simulink model "intgratedMCUSlugs"  (Simulink 7.8)
settings: Solver=FixedStepDiscrete  SolverMode=SingleTasking  StartTime=0.0  StopTime=10.0  FixedStep=0.001  RelTol=1e-3
InitFcn:
  | mcuInit
undefined symbols (not defined in the file): accBiasRateLimit, apSampleTime, barAdjust, baroCutoff, baroCutTemp, baroOffset, baroScale, barTGain1, barTGain2, barTMean1, barTMean2, baseHeight, baseTemp, bda, bde, bdr, bdt, bICda, bICde, bICdr, bICdt, bpan, bPWMpan, bPWMtilt, broll, btilt, changeZoom, controlMCUInit, cubeAccelGain16405, cubeGyroGain16405, cubeMagGain16405, daTrimMax, daTrimMin, deTrimMax, deTrimMin, DiscIntNeverNeededParam, drTrimMax, drTrimMin, dtTrimMax, dtTrimMin, Function_Update, gaind, getCubeData, getGpsMainData, getGPSRawData, getGpsUbloxMainData, getGSLocation, getISRLocation, getMidLevelCommands, getMobileLocation, getPassValues, getRangeOfParams, getRTB, gpsParse, gsRead, gyroBiasRateLimit, hil_getEuler, hil_getRates, hil_getRawRead, hil_getVned ... (+89)
libraries: dsPICdrivers x105, simulink x14, SLUGS_Library x12, aerolibconvert2 x5, aerolibutil x4, aerolibtransform2 x3, dspmtrx3 x3, aerolibobsolete x3
(part 4 of 6)

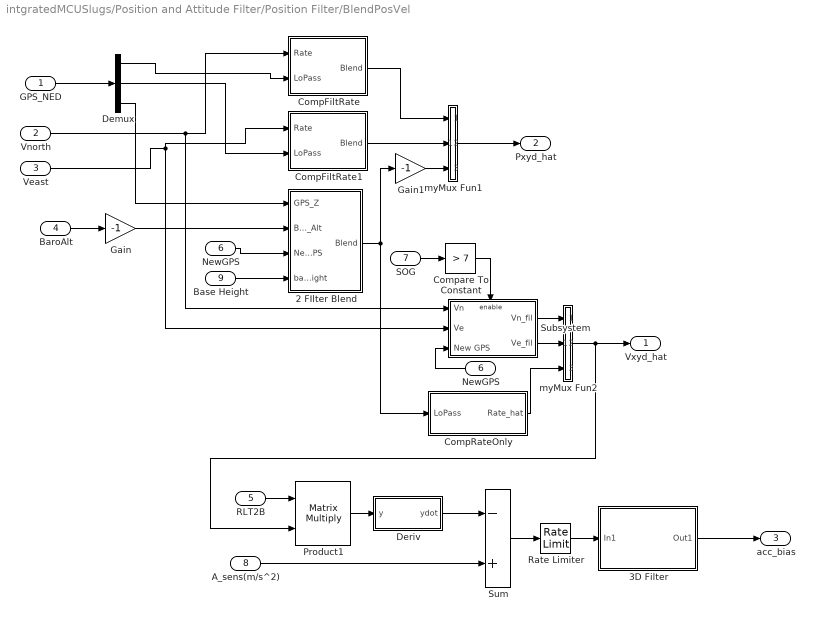
== system intgratedMCUSlugs/Position and Attitude Filter/Position Filter/BlendPosVel ==
  GPS_NED : Inport
  Vnorth : Inport  Port=2
  Veast : Inport  Port=3
  BaroAlt : Inport  Port=4
  RLT2B : Inport  Port=5
  NewGPS : Inport  Port=6
  SOG : Inport  Port=7
  A_sens(m/s^2) : Inport  Port=8
  Base Height : Inport  Port=9
  2 FIlter Blend : Subsystem
  3D Filter : Subsystem  AncestorBlock=SLUGS_Library/Singnal Routing & Conditioning/3D Filter  RTWFcnName=TustinFilter3D  mask{zval=[], pval=-1/accBiasRateLimit, kval=1, TSample=0.01}
      mask prompts: zval "Zeros"; pval "Poles"; kval "Gains"; TSample "Sample Time"
      settings: RTWFcnNameOpts=User specified  RTWFileNameOpts=Use function name
      mask Display:
      | droots(zval,pval,kval)
      | port_label('input',1,'3D')
  CompFiltRate : Subsystem  mask{omega=xCutoff, T=apSampleTime}
      mask prompts: omega "Cutoff Freq (rad/sec)"; T "Sample Time"
  CompFiltRate1 : Subsystem  mask{omega=yCutoff, T=apSampleTime}
      mask prompts: omega "Cutoff Freq (rad/sec)"; T "Sample Time"
  CompRateOnly : Subsystem  mask{omega=vzCutoff, T=apSampleTime}
      mask prompts: omega "Cutoff Freq (rad/sec)"; T "Sample Time"
  Compare To Constant : simulink/Logic and Bit Operations/Compare To Constant  relop=>  const=7  OutDataTypeStr=uint8  ZeroCross=off
  Demux : Demux  Outputs=3
  "Deriv " : Subsystem
  Gain : Gain  Gain=-1
  Gain1 : Gain  Gain=-1  OutDataTypeStr=Inherit: Same as input
  "NewGPS " : InportShadow  Port=6
  Product1 : Product  Multiplication=Matrix(*)  RndMeth=Zero
  Rate Limiter : RateLimiter  RisingSlewLimit=accBiasRateLimit  FallingSlewLimit=-accBiasRateLimit  SampleTimeMode=inherited
  Subsystem : Subsystem
  Sum : Sum  Inputs=-+  OutDataTypeStr=single
  myMux Fun1 : MATLAB Function  TreatAsAtomicUnit=on
  myMux Fun2 : MATLAB Function  TreatAsAtomicUnit=on
  Vxyd_hat : Outport
  Pxyd_hat : Outport  Port=2
  acc_bias : Outport  Port=3
  wires:
  CompRateOnly/1(Rate_hat) -> myMux Fun2/3(u3)
  Subsystem/2(Ve_fil) -> myMux Fun2/2(u2)
  Subsystem/1(Vn_fil) -> myMux Fun2/1(u1)
  myMux Fun1/1(y) -> Pxyd_hat/1
  2 FIlter Blend/1(Blend) -> Gain1/1, CompRateOnly/1(LoPass)
  CompFiltRate/1(Blend) -> myMux Fun1/1(u1)
  CompFiltRate1/1(Blend) -> myMux Fun1/2(u2)
  Demux/3 -> 2 FIlter Blend/1(GPS_Z)
  BaroAlt/1 -> Gain/1
  Demux/2 -> CompFiltRate1/2(LoPass)
  Demux/1 -> CompFiltRate/2(LoPass)
  Veast/1 -> CompFiltRate1/1(Rate), Subsystem/2(Ve)
  Vnorth/1 -> Subsystem/1(Vn), CompFiltRate/1(Rate)
  GPS_NED/1 -> Demux/1
  Gain1/1 -> myMux Fun1/3(u3)
  myMux Fun2/1(y) -> Vxyd_hat/1, Product1/2
  NewGPS/1 -> Subsystem/3(New GPS)
  Compare To Constant/1 -> Subsystem/Enable
  SOG/1 -> Compare To Constant/1
  Rate Limiter/1 -> 3D Filter/1(In1)
  3D Filter/1(Out1) -> acc_bias/1
  Sum/1 -> Rate Limiter/1
  Product1/1 -> "Deriv "/1(y)
  "Deriv "/1(ydot) -> Sum/1
  A_sens(m/s^2)/1 -> Sum/2
  RLT2B/1 -> Product1/1
  Gain/1 -> 2 FIlter Blend/2(Baro_Alt)
  "NewGPS "/1 -> 2 FIlter Blend/3(New GPS)
  Base Height/1 -> 2 FIlter Blend/4(baseHeight)

== system intgratedMCUSlugs/Sensor Data/Sensor Suite/ADIS16405 Signal Cond  ==
  Gyro Raw : Inport
  Accel Raw : Inport  Port=2
  Mag Raw : Inport  Port=3
  "3D Tustin Lowpass, Auto Initial Condition" : Subsystem  mask(Tustin1stOrderLowpassAutoInitialCondition){f=mainSensorCutoff, T=T}
      mask prompts: f "Lowpass Frequency"; T "Sample Time"
      mask help: Takes a 3db rolloff frequency (in Hz, NOT radians/s) and a sample time. Performs a symbolic Tustin conversion and implements in a discrete filter. The initial output of the filter is set by the first sample.
      mask Help: Enter the desired 3db rolloff frequency in Hz and the sample time. Initial conditions are sampled automatically.
      mask Display: fprintf('%.2f Hz lowpass (3D)',f)
  "3D Tustin Lowpass, Auto Initial Condition1" : Subsystem  mask(Tustin1stOrderLowpassAutoInitialCondition){f=mainSensorCutoff, T=T}
      mask prompts: f "Lowpass Frequency"; T "Sample Time"
      mask help: Takes a 3db rolloff frequency (in Hz, NOT radians/s) and a sample time. Performs a symbolic Tustin conversion and implements in a discrete filter. The initial output of the filter is set by the first sample.
      mask Help: Enter the desired 3db rolloff frequency in Hz and the sample time. Initial conditions are sampled automatically.
      mask Display: fprintf('%.2f Hz lowpass (3D)',f)
  "3D Tustin Lowpass, Auto Initial Condition2" : Subsystem  mask(Tustin1stOrderLowpassAutoInitialCondition){f=mainSensorCutoff, T=T}
      mask prompts: f "Lowpass Frequency"; T "Sample Time"
      mask help: Takes a 3db rolloff frequency (in Hz, NOT radians/s) and a sample time. Performs a symbolic Tustin conversion and implements in a discrete filter. The initial output of the filter is set by the first sample.
      mask Help: Enter the desired 3db rolloff frequency in Hz and the sample time. Initial conditions are sampled automatically.
      mask Display: fprintf('%.2f Hz lowpass (3D)',f)
  Data Type Conversion1 : DataTypeConversion  OutDataTypeStr=double
  Data Type Conversion2 : DataTypeConversion  OutDataTypeStr=double
  Data Type Conversion3 : DataTypeConversion  OutDataTypeStr=single
  Data Type Conversion5 : DataTypeConversion  OutDataTypeStr=double
  Data Type Conversion6 : DataTypeConversion  OutDataTypeStr=single
  Data Type Conversion7 : DataTypeConversion  OutDataTypeStr=single
  Divide : Product  OutDataTypeStr=single
  Divide1 : Product  OutDataTypeStr=single
  Divide2 : Product  OutDataTypeStr=single
  Gyro Gains : Constant  Value=cubeGyroGain16405  OutDataTypeStr=single
  Gyro Gains1 : Constant  Value=cubeAccelGain16405  OutDataTypeStr=single
  Gyro Gains2 : Constant  Value=cubeMagGain16405  OutDataTypeStr=single
  Rotate Cube Axis : Subsystem
  "Rotate Cube Axis " : Subsystem
  "Rotate Cube Axis  " : Subsystem
  Omega (rad/s) : Outport
  Accel (m/s^2) : Outport  Port=2
  Mags (mG) : Outport  Port=3
  wires:
  Gyro Gains/1 -> Divide/2
  Divide/1 -> Rotate Cube Axis/1(Raw)
  Divide1/1 -> "Rotate Cube Axis "/1(Raw)
  "Rotate Cube Axis "/1(Rotated) -> Data Type Conversion1/1
  Gyro Gains1/1 -> Divide1/2
  Gyro Raw/1 -> Divide/1
  Data Type Conversion2/1 -> "3D Tustin Lowpass, Auto Initial Condition"/1(In1)
  "3D Tustin Lowpass, Auto Initial Condition"/1(Out1) -> Data Type Conversion7/1
  Data Type Conversion7/1 -> Omega (rad/s)/1
  Rotate Cube Axis/1(Rotated) -> Data Type Conversion2/1
  Data Type Conversion1/1 -> "3D Tustin Lowpass, Auto Initial Condition1"/1(In1)
  "3D Tustin Lowpass, Auto Initial Condition1"/1(Out1) -> Data Type Conversion3/1
  Data Type Conversion3/1 -> Accel (m/s^2)/1
  Accel Raw/1 -> Divide1/1
  Divide2/1 -> "Rotate Cube Axis  "/1(Raw)
  Data Type Conversion5/1 -> "3D Tustin Lowpass, Auto Initial Condition2"/1(In1)
  "3D Tustin Lowpass, Auto Initial Condition2"/1(Out1) -> Data Type Conversion6/1
  Data Type Conversion6/1 -> Mags (mG)/1
  "Rotate Cube Axis  "/1(Rotated) -> Data Type Conversion5/1
  Mag Raw/1 -> Divide2/1
  Gyro Gains2/1 -> Divide2/2

== system intgratedMCUSlugs/Sensor Data/Sensor Suite/Compute CPU Load ==
  Calculus Time Step : dsPICdrivers/OTHERS/Calculus Time Step  Tag=dsPIC_CalculusTimeStep  SampleTime=0.01  PR1chk=on
  Constant : Constant
  Data Type Conversion1 : DataTypeConversion  OutDataTypeStr=single
  Data Type Conversion12 : DataTypeConversion  OutDataTypeStr=uint8
  Data Type Conversion2 : DataTypeConversion  OutDataTypeStr=single
  Divide : Product  Inputs=*/  OutDataTypeStr=double
  Gain : Gain  Gain=100
  Rounding Function : Rounding
  Switch : Switch  Criteria=u2 > Threshold
  Load (%) : Outport
  wires:
  Calculus Time Step/1 -> Data Type Conversion2/1
  Calculus Time Step/2 -> Data Type Conversion1/1
  Divide/1 -> Gain/1
  Rounding Function/1 -> Data Type Conversion12/1
  Data Type Conversion2/1 -> Divide/1
  Data Type Conversion12/1 -> Load (%)/1
  Gain/1 -> Rounding Function/1
  Data Type Conversion1/1 -> Switch/2, Switch/1
  Constant/1 -> Switch/3
  Switch/1 -> Divide/2

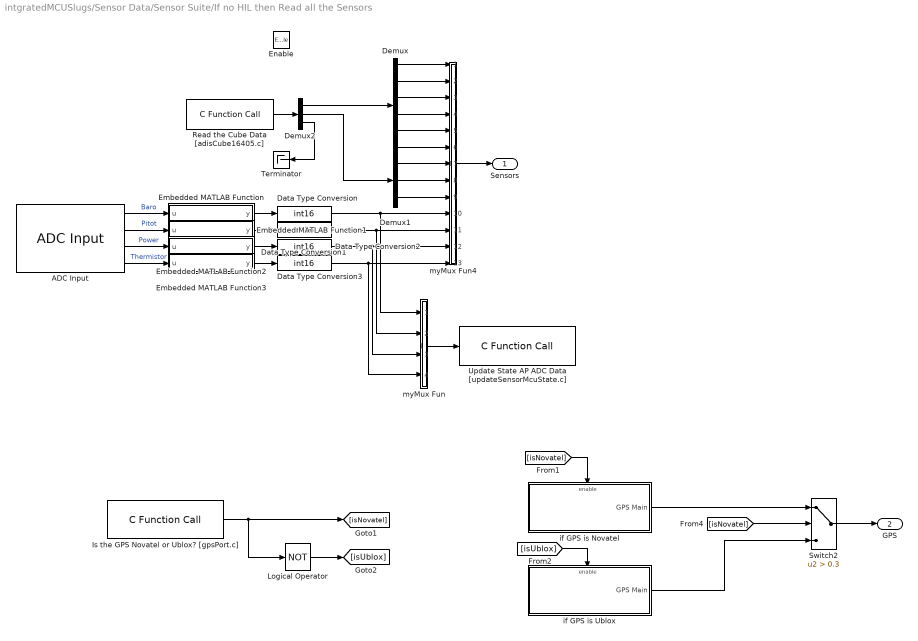
== system intgratedMCUSlugs/Sensor Data/Sensor Suite/If no HIL then Read all the Sensors ==
  Enable : EnablePort
  ADC Input : dsPICdrivers/Peripheral I//O/ADC Input  Tag=dsPIC_ADC  Priority=5  ADC_TYPE=12 bits  ADC_MODE=Continuous sampling & get last channel value  NbrSampleStep=5  VoltRefpopup="AVdd  -  AVss"  OutFormatBitspopup=0000 dddd dddd dddd : Integer  InterruptPriority=6  ANCHANNELS=[8 9 10 11]  MaxName=ANmax = 4095  Rin=200  ADCS=63  SAMC=31  Temperature=25  DMAChannel=1  SampleTime=.01  Status="OK  |  Tsmp=2.480e-005 |  T/Channel=3.600e-005 |  Tall=7.200e-004"  SSRC=auto convert
  Data Type Conversion{,1..3} (4 alike) : DataTypeConversion  OutDataTypeStr=int16
  Demux : Demux  Outputs=6
  Demux1 : Demux  Outputs=3
  Demux2 : Demux  Outputs=[6 3 1]
  Embedded MATLAB Function : MATLAB Function  TreatAsAtomicUnit=on
  Embedded MATLAB Function1 : MATLAB Function  TreatAsAtomicUnit=on
  Embedded MATLAB Function2 : MATLAB Function  TreatAsAtomicUnit=on
  Embedded MATLAB Function3 : MATLAB Function  TreatAsAtomicUnit=on
  Is the GPS Novatel or Ublox? [gpsPort.c] : dsPICdrivers/OTHERS/C Function Call  Tag=dsPIC_dsPIC_CFunctionCall  FctUpdate=Output Function  fctName='isGPSNovatel'  INPUT_SIZE=1  INPUT1=--  INPUT2=--  INPUT3=--  OUTPUT_SIZE=1  OUTPUT1=uint8  SampleTime=.01  InputType=[ ]  OutputType=[ 2 ]  FctDeclaration=extern uint8_T isGPSNovatel();  FctCall=%y1 = isGPSNovatel();  OrderingInOutPopup=None  FctStart=None  FctStart_Name=Init_onlyOnce  FctStart_Declaration=inline extern void Init_onlyOnce();  FctStart_Call=Init_onlyOnce();  FctInit=None  FctInit_Name=Init_Reset  FctInit_Declaration=inline extern void Init_Reset();  FctInit_Call=Init_Reset();  PinDigitalInput=[]  PinDigitalOutput=[]  AnalogueInput=[]
  Logical Operator : Logic  Operator=NOT  AllPortsSameDT=off  OutDataTypeStr=boolean
  Read the Cube Data [adisCube16405.c] : dsPICdrivers/OTHERS/C Function Call  Tag=dsPIC_dsPIC_CFunctionCall  FctUpdate=Output Function  fctName='getCubeData'  INPUT_SIZE=1  INPUT1=--  INPUT2=--  INPUT3=--  OUTPUT_SIZE=10  OUTPUT1=int16  SampleTime=.01  InputType=[ ]  OutputType=[ 3 ]  FctDeclaration=extern void getCubeData(int16_T* y1);  FctCall=getCubeData(*%y1);  OrderingInOutPopup=None  FctStart=None  FctStart_Name=Init_onlyOnce  FctStart_Declaration=inline extern void Init_onlyOnce();  FctStart_Call=Init_onlyOnce();  FctInit=None  FctInit_Name=Init_Reset  FctInit_Declaration=inline extern void Init_Reset();  FctInit_Call=Init_Reset();  PinDigitalInput=[]  PinDigitalOutput=[]  AnalogueInput=[]
  Switch2 : Switch  Criteria=u2 > Threshold  Threshold=0.3  ZeroCross=off
  Terminator : Terminator
  Update State AP ADC Data [updateSensorMcuState.c] : dsPICdrivers/OTHERS/C Function Call  Tag=dsPIC_dsPIC_CFunctionCall  FctUpdate=Output Function  fctName='updateRawADCData'  INPUT_SIZE=4  INPUT1=int16  INPUT2=--  INPUT3=--  OUTPUT_SIZE=1  OUTPUT1=--  SampleTime=.01  InputType=[ 3 ]  OutputType=[ ]  FctDeclaration=extern void updateRawADCData(int16_T* u1);  FctCall=updateRawADCData(*%u1);  OrderingInOutPopup=None  FctStart=None  FctStart_Name=Init_onlyOnce  FctStart_Declaration=inline extern void Init_onlyOnce();  FctStart_Call=Init_onlyOnce();  FctInit=None  FctInit_Name=Init_Reset  FctInit_Declaration=inline extern void Init_Reset();  FctInit_Call=Init_Reset();  PinDigitalInput=[]  PinDigitalOutput=[]  AnalogueInput=[]
  if GPS is Novatel : Subsystem
  if GPS is Ublox : Subsystem
  myMux Fun : MATLAB Function  TreatAsAtomicUnit=on
  myMux Fun4 : MATLAB Function  TreatAsAtomicUnit=on
  Sensors : Outport
  GPS : Outport  Port=2
  wires:
  myMux Fun4/1(y) -> Sensors/1
  Demux2/1 -> Demux/1
  Demux/1 -> myMux Fun4/1(u1)
  Demux/2 -> myMux Fun4/2(u2)
  Demux/3 -> myMux Fun4/3(u3)
  Demux/4 -> myMux Fun4/4(u4)
  Demux/5 -> myMux Fun4/5(u5)
  Demux/6 -> myMux Fun4/6(u6)
  Demux1/1 -> myMux Fun4/7(u7)
  Demux1/2 -> myMux Fun4/8(u8)
  Demux1/3 -> myMux Fun4/9(u9)
  ADC Input/1 -> Embedded MATLAB Function/1(u)  "Baro"
  ADC Input/2 -> Embedded MATLAB Function1/1(u)  "Pitot"
  ADC Input/3 -> Embedded MATLAB Function2/1(u)  "Power"
  ADC Input/4 -> Embedded MATLAB Function3/1(u)  "Thermistor"
  myMux Fun/1(y) -> Update State AP ADC Data [updateSensorMcuState.c]/1
  Data Type Conversion/1 -> myMux Fun4/10(u10), myMux Fun/1(u1)
  Data Type Conversion1/1 -> myMux Fun4/11(u11), myMux Fun/2(u2)
  Data Type Conversion2/1 -> myMux Fun4/12(u12), myMux Fun/3(u3)
  Data Type Conversion3/1 -> myMux Fun4/13(u13), myMux Fun/4(u4)
  Embedded MATLAB Function/1(y) -> Data Type Conversion/1
  Embedded MATLAB Function1/1(y) -> Data Type Conversion1/1
  Embedded MATLAB Function2/1(y) -> Data Type Conversion2/1
  Embedded MATLAB Function3/1(y) -> Data Type Conversion3/1
  Read the Cube Data [adisCube16405.c]/1 -> Demux2/1
  Demux2/3 -> Terminator/1
  Demux2/2 -> Demux1/1
  [isNovatel] -> Switch2/2
  Switch2/1 -> GPS/1
  Is the GPS Novatel or Ublox? [gpsPort.c]/1 -> [isNovatel], Logical Operator/1
  if GPS is Novatel/1(GPS Main) -> Switch2/1
  Logical Operator/1 -> [isUblox]
  [isNovatel] -> if GPS is Novatel/Enable
  [isUblox] -> if GPS is Ublox/Enable
  if GPS is Ublox/1(GPS Main) -> Switch2/3

== system intgratedMCUSlugs/Sensor Data/Sensor Suite/If no HIL then update Air Data ==
  AirData : Inport
  Enable : EnablePort
  Demux : Demux  Outputs=[1 2]
  Terminator : Terminator
  Update the Air Calibrated Data [updateSensorMcuState.c] : dsPICdrivers/OTHERS/C Function Call  Tag=dsPIC_dsPIC_CFunctionCall  FctUpdate=Output Function  fctName='updateAirData'  INPUT_SIZE=3  INPUT1=real32  INPUT2=--  INPUT3=--  OUTPUT_SIZE=1  OUTPUT1=--  SampleTime=.01  InputType=[ 7 ]  OutputType=[ ]  FctDeclaration=extern void updateAirData(real32_T* u1);  FctCall=updateAirData(*%u1);  OrderingInOutPopup=None  FctStart=None  FctStart_Name=Init_onlyOnce  FctStart_Declaration=inline extern void Init_onlyOnce();  FctStart_Call=Init_onlyOnce();  FctInit=None  FctInit_Name=Init_Reset  FctInit_Declaration=inline extern void Init_Reset();  FctInit_Call=Init_Reset();  PinDigitalInput=[]  PinDigitalOutput=[]  AnalogueInput=[]
  Out1 : Outport
  wires:
  AirData/1 -> Update the Air Calibrated Data [updateSensorMcuState.c]/1, Demux/1
  Demux/1 -> Out1/1
  Demux/2 -> Terminator/1

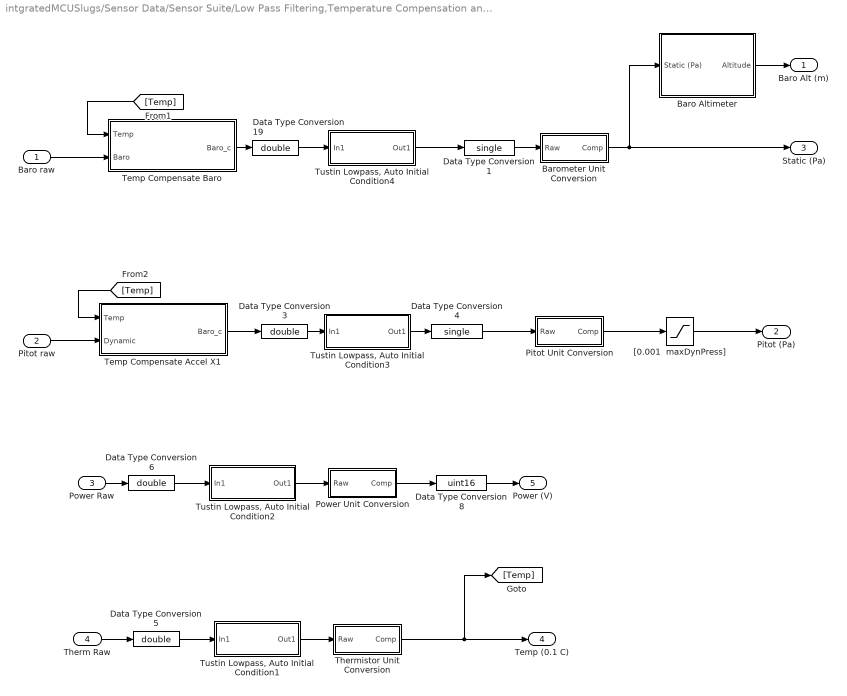
== system intgratedMCUSlugs/Sensor Data/Sensor Suite/Low Pass Filtering,Temperature Compensation and Calibration ==
  Baro raw : Inport
  Pitot raw : Inport  Port=2
  Power Raw : Inport  Port=3
  Therm Raw : Inport  Port=4
  Baro Altimeter : Subsystem
  Barometer Unit Conversion : Subsystem  mask{bias=baroOffset, gains=baroScale}
      mask prompts: bias "Initial Bias"; gains "Initial Gains"
      mask help: Convert Analog readings to units
  Data Type Conversion1 : DataTypeConversion  OutDataTypeStr=single
  Data Type Conversion{3,5..6,19} (4 alike) : DataTypeConversion  OutDataTypeStr=double
  Data Type Conversion4 : DataTypeConversion  OutDataTypeStr=single
  Data Type Conversion8 : DataTypeConversion  OutDataTypeStr=uint16
  Pitot Unit Conversion : Subsystem  mask{bias=pitotOffset, gains=pitotScale}
      mask prompts: bias "Initial Bias"; gains "Initial Gains"
      mask help: Convert Analog readings to units
  Power Unit Conversion : Subsystem  mask{bias=powerOffset, gains=powerScale}
      mask prompts: bias "Initial Bias"; gains "Initial Gains"
      mask help: Convert Analog readings to units
  Temp Compensate Accel X1 : Subsystem
  Temp Compensate Baro : Subsystem
  Thermistor Unit Conversion : Subsystem  mask{bias=tempOffset, gains=tempScale}
      mask prompts: bias "Initial Bias"; gains "Initial Gains"
      mask help: Convert Analog readings to units
  "Tustin Lowpass, Auto Initial Condition1" : Subsystem  mask(Tustin1stOrderLowpassAutoInitialCondition){f=lowRateSensorCutoff, T=apSampleTime}
      mask prompts: f "Lowpass Frequency"; T "Sample Time"
      mask help: Takes a 3db rolloff frequency (in Hz, NOT radians/s) and a sample time. Performs a symbolic Tustin conversion and implements in a discrete filter. The initial output of the filter is set by the first sample.
      mask Help: Enter the desired 3db rolloff frequency in Hz and the sample time. Initial conditions are sampled automatically.
      mask Display: fprintf('%.2f Hz lowpass',f)
  "Tustin Lowpass, Auto Initial Condition2" : Subsystem  mask(Tustin1stOrderLowpassAutoInitialCondition){f=lowRateSensorCutoff, T=apSampleTime}
      mask prompts: f "Lowpass Frequency"; T "Sample Time"
      mask help: Takes a 3db rolloff frequency (in Hz, NOT radians/s) and a sample time. Performs a symbolic Tustin conversion and implements in a discrete filter. The initial output of the filter is set by the first sample.
      mask Help: Enter the desired 3db rolloff frequency in Hz and the sample time. Initial conditions are sampled automatically.
      mask Display: fprintf('%.2f Hz lowpass',f)
  "Tustin Lowpass, Auto Initial Condition3" : Subsystem  mask(Tustin1stOrderLowpassAutoInitialCondition){f=pressureSensorCutoff, T=apSampleTime}
      mask prompts: f "Lowpass Frequency"; T "Sample Time"
      mask help: Takes a 3db rolloff frequency (in Hz, NOT radians/s) and a sample time. Performs a symbolic Tustin conversion and implements in a discrete filter. The initial output of the filter is set by the first sample.
      mask Help: Enter the desired 3db rolloff frequency in Hz and the sample time. Initial conditions are sampled automatically.
      mask Display: fprintf('%.2f Hz lowpass',f)
  "Tustin Lowpass, Auto Initial Condition4" : Subsystem  mask(Tustin1stOrderLowpassAutoInitialCondition){f=pressureSensorCutoff, T=apSampleTime}
      mask prompts: f "Lowpass Frequency"; T "Sample Time"
      mask help: Takes a 3db rolloff frequency (in Hz, NOT radians/s) and a sample time. Performs a symbolic Tustin conversion and implements in a discrete filter. The initial output of the filter is set by the first sample.
      mask Help: Enter the desired 3db rolloff frequency in Hz and the sample time. Initial conditions are sampled automatically.
      mask Display: fprintf('%.2f Hz lowpass',f)
  "[0.001  maxDynPress]" : Saturate  UpperLimit=maxDynPressure  LowerLimit=0.001
  Baro Alt (m) : Outport
  Pitot (Pa) : Outport  Port=2
  Static (Pa) : Outport  Port=3
  Temp (0.1 C) : Outport  Port=4
  Power (V) : Outport  Port=5
  wires:
  "Tustin Lowpass, Auto Initial Condition1"/1(Out1) -> Thermistor Unit Conversion/1(Raw)
  "[0.001  maxDynPress]"/1 -> Pitot (Pa)/1
  Data Type Conversion19/1 -> "Tustin Lowpass, Auto Initial Condition4"/1(In1)
  Data Type Conversion3/1 -> "Tustin Lowpass, Auto Initial Condition3"/1(In1)
  "Tustin Lowpass, Auto Initial Condition3"/1(Out1) -> Data Type Conversion4/1
  Data Type Conversion5/1 -> "Tustin Lowpass, Auto Initial Condition1"/1(In1)
  Therm Raw/1 -> Data Type Conversion5/1
  Barometer Unit Conversion/1(Comp) -> Static (Pa)/1, Baro Altimeter/1(Static (Pa))
  Data Type Conversion4/1 -> Pitot Unit Conversion/1(Raw)
  "Tustin Lowpass, Auto Initial Condition4"/1(Out1) -> Data Type Conversion1/1
  Data Type Conversion1/1 -> Barometer Unit Conversion/1(Raw)
  Thermistor Unit Conversion/1(Comp) -> Temp (0.1 C)/1, [Temp]
  Data Type Conversion6/1 -> "Tustin Lowpass, Auto Initial Condition2"/1(In1)
  Power Raw/1 -> Data Type Conversion6/1
  "Tustin Lowpass, Auto Initial Condition2"/1(Out1) -> Power Unit Conversion/1(Raw)
  Data Type Conversion8/1 -> Power (V)/1
  Baro Altimeter/1(Altitude) -> Baro Alt (m)/1
  Pitot Unit Conversion/1(Comp) -> "[0.001  maxDynPress]"/1
  Power Unit Conversion/1(Comp) -> Data Type Conversion8/1
  Temp Compensate Baro/1(Baro_c) -> Data Type Conversion19/1
  [Temp] -> Temp Compensate Baro/1(Temp)
  Baro raw/1 -> Temp Compensate Baro/2(Baro)
  [Temp] -> Temp Compensate Accel X1/1(Temp)
  Pitot raw/1 -> Temp Compensate Accel X1/2(Dynamic)
  Temp Compensate Accel X1/1(Baro_c) -> Data Type Conversion3/1

== system intgratedMCUSlugs/Trim Vals/Control Surface Input/2 sec  tau ==
  In1 : Inport
  Constant : Constant  Value=T
  Constant1 : Constant  Value=f
  Embedded MATLAB Function : MATLAB Function  TreatAsAtomicUnit=on
  Out1 : Outport
  wires:
  In1/1 -> Embedded MATLAB Function/1(u)
  Embedded MATLAB Function/1(y) -> Out1/1
  Constant1/1 -> Embedded MATLAB Function/3(f)
  Constant/1 -> Embedded MATLAB Function/2(T)

== system intgratedMCUSlugs/Trim Vals/Control Surface Input/2 sec  tau1 ==
  In1 : Inport
  Constant : Constant  Value=T
  Constant1 : Constant  Value=f
  Embedded MATLAB Function : MATLAB Function  TreatAsAtomicUnit=on
  Out1 : Outport
  wires:
  Constant/1 -> Embedded MATLAB Function/2(T)
  Constant1/1 -> Embedded MATLAB Function/3(f)
  Embedded MATLAB Function/1(y) -> Out1/1
  In1/1 -> Embedded MATLAB Function/1(u)

== system intgratedMCUSlugs/Trim Vals/Detect Transition High to Low/Subsystem ==
  WP Fly : Inport
  Data Type Conversion1 : DataTypeConversion  OutDataTypeStr=uint8  SampleTime=apSampleTime
  Detect Rising Transition [navSupport.c] : dsPICdrivers/OTHERS/C Function Call  Tag=dsPIC_dsPIC_CFunctionCall  FctUpdate=Output Function  fctName='justEnabled'  INPUT_SIZE=1  INPUT1=uint8  INPUT2=uint8  INPUT3=--  OUTPUT_SIZE=1  OUTPUT1=uint8  SampleTime=0.01  InputType=[ 2 2 ]  OutputType=[ 2 ]  FctDeclaration=extern uint8_T justEnabled(uint8_T u1, uint8_T u2);  FctCall=%y1 = justEnabled(%u1, %u2);  OrderingInOutPopup=None  FctStart=None  FctStart_Name=Init_onlyOnce  FctStart_Declaration=inline extern void Init_onlyOnce();  FctStart_Call=Init_onlyOnce();  FctInit=None  FctInit_Name=Init_Reset  FctInit_Declaration=inline extern void Init_Reset();  FctInit_Call=Init_Reset();  PinDigitalInput=[]  PinDigitalOutput=[]  AnalogueInput=[]
  Index : Constant  Value=2  OutDataTypeStr=uint8
  Just Enab : Outport
  wires:
  Detect Rising Transition [navSupport.c]/1 -> Just Enab/1
  WP Fly/1 -> Data Type Conversion1/1
  Data Type Conversion1/1 -> Detect Rising Transition [navSupport.c]/1
  Index/1 -> Detect Rising Transition [navSupport.c]/2

== system intgratedMCUSlugs/Trim Vals/Grab I.C./Convert to Microseconds  ==
  IC : Inport
  Convert to  Microseconds : Gain  Gain=0.2
  Data Type Conversion : DataTypeConversion  OutDataTypeStr=uint16
  uS : Outport
  wires:
  Convert to  Microseconds/1 -> Data Type Conversion/1
  IC/1 -> Convert to  Microseconds/1
  Data Type Conversion/1 -> uS/1

== system intgratedMCUSlugs/Trim Vals/Grab I.C./Convert to Microseconds 1 ==
  IC : Inport
  Convert to  Microseconds : Gain  Gain=0.2
  Data Type Conversion : DataTypeConversion  OutDataTypeStr=uint16
  uS : Outport
  wires:
  Data Type Conversion/1 -> uS/1
  IC/1 -> Convert to  Microseconds/1
  Convert to  Microseconds/1 -> Data Type Conversion/1

== system intgratedMCUSlugs/Trim Vals/Grab I.C./Convert to Microseconds 2 ==
  IC : Inport
  Convert to  Microseconds : Gain  Gain=0.2
  Data Type Conversion : DataTypeConversion  OutDataTypeStr=uint16
  uS : Outport
  wires:
  Convert to  Microseconds/1 -> Data Type Conversion/1
  IC/1 -> Convert to  Microseconds/1
  Data Type Conversion/1 -> uS/1

== system intgratedMCUSlugs/Trim Vals/Grab I.C./Convert to Microseconds 3 ==
  IC : Inport
  Convert to  Microseconds : Gain  Gain=0.2
  Data Type Conversion : DataTypeConversion  OutDataTypeStr=uint16
  uS : Outport
  wires:
  Data Type Conversion/1 -> uS/1
  IC/1 -> Convert to  Microseconds/1
  Convert to  Microseconds/1 -> Data Type Conversion/1

== system intgratedMCUSlugs/Trim Vals/Grab I.C./Convert to Rad ==
  IC : Inport
  Add : Sum
  Constant1 : Constant  Value=slopem
  Constant2 : Constant  Value=interceptb
  Data Type Conversion : DataTypeConversion  OutDataTypeStr=single
  Divide : Product
  Angle (rad) : Outport
  wires:
  Data Type Conversion/1 -> Angle (rad)/1
  IC/1 -> Divide/1
  Constant2/1 -> Add/2
  Divide/1 -> Add/1
  Add/1 -> Data Type Conversion/1
  Constant1/1 -> Divide/2

== system intgratedMCUSlugs/Trim Vals/Grab I.C./Convert to Rad1 ==
  IC : Inport
  Add : Sum
  Constant1 : Constant  Value=slopem
  Constant2 : Constant  Value=interceptb
  Data Type Conversion : DataTypeConversion  OutDataTypeStr=single
  Divide : Product
  Angle (rad) : Outport
  wires:
  Constant1/1 -> Divide/2
  Add/1 -> Data Type Conversion/1
  Divide/1 -> Add/1
  Constant2/1 -> Add/2
  IC/1 -> Divide/1
  Data Type Conversion/1 -> Angle (rad)/1

== system intgratedMCUSlugs/Trim Vals/Grab I.C./Convert to Rad2 ==
  IC : Inport
  Add : Sum
  Constant1 : Constant  Value=slopem
  Constant2 : Constant  Value=interceptb
  Data Type Conversion : DataTypeConversion  OutDataTypeStr=single
  Divide : Product
  Angle (rad) : Outport
  wires:
  Data Type Conversion/1 -> Angle (rad)/1
  IC/1 -> Divide/1
  Constant2/1 -> Add/2
  Divide/1 -> Add/1
  Add/1 -> Data Type Conversion/1
  Constant1/1 -> Divide/2

== system intgratedMCUSlugs/Trim Vals/Grab I.C./Convert to Rad3 ==
  IC : Inport
  Add : Sum
  Constant1 : Constant  Value=slopem
  Constant2 : Constant  Value=interceptb
  Data Type Conversion : DataTypeConversion  OutDataTypeStr=single
  Divide : Product
  Angle (rad) : Outport
  wires:
  Constant1/1 -> Divide/2
  Add/1 -> Data Type Conversion/1
  Divide/1 -> Add/1
  Constant2/1 -> Add/2
  IC/1 -> Divide/1
  Data Type Conversion/1 -> Angle (rad)/1

== system intgratedMCUSlugs/Update PWM Commands and Send Telemetry/Generate PWM Signals Based on the Control Type/If  Control Type Is Manual ==
  Pilot (IC) : Inport
  Action Port : ActionPort  ActionType=then
  Gain4 : Gain  Gain=0.5  OutDataTypeStr=Inherit: Same as input
  PWM : Outport
  wires:
  Pilot (IC)/1 -> Gain4/1
  Gain4/1 -> PWM/1

== system intgratedMCUSlugs/Update PWM Commands and Send Telemetry/Generate PWM Signals Based on the Control Type/If  Control Type Is Passthrough ==
  Pilot (IC) : Inport
  Action Port : ActionPort  ActionType=elseif
  Gain4 : Gain  Gain=0.5  OutDataTypeStr=Inherit: Same as input
  PWM (abs) : Outport
  wires:
  Gain4/1 -> PWM (abs)/1
  Pilot (IC)/1 -> Gain4/1

== system intgratedMCUSlugs/Update PWM Commands and Send Telemetry/Generate PWM Signals Based on the Control Type/If  Control Type Is Selective Passthrough ==
  PWM(rad) : Inport
  Pilot (IC) : Inport  Port=2
  Action Port : ActionPort  ActionType=elseif
  Convert to PWM : Subsystem  mask{slopem=mde, interceptb=bde}
      mask prompts: slopem "Slope"; interceptb "Intercept"
  Convert to PWM1 : Subsystem  mask{slopem=mdt, interceptb=bdt}
      mask prompts: slopem "Slope"; interceptb "Intercept"
  Convert to PWM2 : Subsystem  mask{slopem=mda, interceptb=bda}
      mask prompts: slopem "Slope"; interceptb "Intercept"
  Convert to PWM3 : Subsystem  mask{slopem=mdr, interceptb=bdr}
      mask prompts: slopem "Slope"; interceptb "Intercept"
  Demux : Demux
  Demux1 : Demux
  Demux2 : Demux
  Gain{,1..3} (4 alike) : Gain  Gain=0.5  OutDataTypeStr=Inherit: Same as input
  Get Pass Switches [navSupport.c] : dsPICdrivers/OTHERS/C Function Call  Tag=dsPIC_dsPIC_CFunctionCall  FctUpdate=Output Function  fctName='getPassValues'  INPUT_SIZE=1  INPUT1=--  INPUT2=--  INPUT3=--  OUTPUT_SIZE=4  OUTPUT1=uint8  SampleTime=.01  InputType=[ ]  OutputType=[ 2 ]  FctDeclaration=extern void getPassValues(uint8_T* y1);  FctCall=getPassValues(*%y1);  OrderingInOutPopup=None  FctStart=None  FctStart_Name=Init_onlyOnce  FctStart_Declaration=inline extern void Init_onlyOnce();  FctStart_Call=Init_onlyOnce();  FctInit=None  FctInit_Name=Init_Reset  FctInit_Declaration=inline extern void Init_Reset();  FctInit_Call=Init_Reset();  PinDigitalInput=[]  PinDigitalOutput=[]  AnalogueInput=[]
  Switch{,1..3} (4 alike) : Switch  Threshold=0.5
  myMux Fun1 : MATLAB Function  TreatAsAtomicUnit=on
  PWM : Outport
  wires:
  myMux Fun1/1(y) -> PWM/1
  Switch/1 -> myMux Fun1/1(u1)
  Switch1/1 -> myMux Fun1/2(u2)
  Switch2/1 -> myMux Fun1/3(u3)
  Switch3/1 -> myMux Fun1/4(u4)
  Get Pass Switches [navSupport.c]/1 -> Demux/1
  Demux/4 -> Switch/2
  Demux/3 -> Switch1/2
  Demux/2 -> Switch2/2
  Demux/1 -> Switch3/2
  Demux1/1 -> Convert to PWM1/1(" Angle(rad)")
  Demux1/2 -> Convert to PWM2/1(" Angle(rad)")
  Demux1/3 -> Convert to PWM3/1(" Angle(rad)")
  Demux1/4 -> Convert to PWM/1(" Angle(rad)")
  PWM(rad)/1 -> Demux1/1
  Convert to PWM1/1(PWM) -> Switch/3
  Convert to PWM2/1(PWM) -> Switch1/3
  Convert to PWM3/1(PWM) -> Switch2/3
  Convert to PWM/1(PWM) -> Switch3/3
  Demux2/1 -> Gain/1
  Demux2/2 -> Gain1/1
  Demux2/3 -> Gain2/1
  Demux2/4 -> Gain3/1
  Pilot (IC)/1 -> Demux2/1
  Gain/1 -> Switch/1
  Gain1/1 -> Switch1/1
  Gain2/1 -> Switch2/1
  Gain3/1 -> Switch3/1

== system intgratedMCUSlugs/Update PWM Commands and Send Telemetry/Generate PWM Signals Based on the Control Type/If  Control Type Is Wp, ISR, LP or  Mid Lvl Cmds ==
  PWM(rad) : Inport
  Action Port : ActionPort  ActionType=elseif
  Convert to PWM : Subsystem  mask{slopem=mde, interceptb=bde}
      mask prompts: slopem "Slope"; interceptb "Intercept"
  Convert to PWM1 : Subsystem  mask{slopem=mdt, interceptb=bdt}
      mask prompts: slopem "Slope"; interceptb "Intercept"
  Convert to PWM2 : Subsystem  mask{slopem=mda, interceptb=bda}
      mask prompts: slopem "Slope"; interceptb "Intercept"
  Convert to PWM3 : Subsystem  mask{slopem=mdr, interceptb=bdr}
      mask prompts: slopem "Slope"; interceptb "Intercept"
  Demux : Demux
  myMux Fun1 : MATLAB Function  TreatAsAtomicUnit=on
  PWM (abs) : Outport
  wires:
  myMux Fun1/1(y) -> PWM (abs)/1
  Convert to PWM1/1(PWM) -> myMux Fun1/1(u1)
  Convert to PWM2/1(PWM) -> myMux Fun1/2(u2)
  Convert to PWM3/1(PWM) -> myMux Fun1/3(u3)
  Convert to PWM/1(PWM) -> myMux Fun1/4(u4)
  Demux/1 -> Convert to PWM1/1(" Angle(rad)")
  Demux/2 -> Convert to PWM2/1(" Angle(rad)")
  Demux/3 -> Convert to PWM3/1(" Angle(rad)")
  Demux/4 -> Convert to PWM/1(" Angle(rad)")
  PWM(rad)/1 -> Demux/1

== system intgratedMCUSlugs/Update PWM Commands and Send Telemetry/PTZ Unit/Camera Stab ==
  Euler : Inport
  Enable : EnablePort
  Add : Sum  Inputs=+-+
  Constant : Constant  Value=0
  Convert to PWM3 : Subsystem  mask{slopem=mtilt, interceptb=btilt}
      mask prompts: slopem "Slope"; interceptb "Intercept"
  Currently No Roll  Comp : Constant  Value=0
  Demux1 : Demux  Outputs=3
  Gain2 : Gain  Gain=-1
  Get the Pan [FCBEX1000.c] : dsPICdrivers/OTHERS/C Function Call  Tag=dsPIC_dsPIC_CFunctionCall  FctUpdate=Output Function  fctName='getPanValue'  INPUT_SIZE=1  INPUT1=uint8  INPUT2=--  INPUT3=--  OUTPUT_SIZE=1  OUTPUT1=uint16  SampleTime=0.01  InputType=[ 2 ]  OutputType=[ 4 ]  FctDeclaration=extern uint16_T getPanValue(uint8_T u1);  FctCall=%y1 = getPanValue(%u1);  OrderingInOutPopup=None  FctStart=None  FctStart_Name=Init_onlyOnce  FctStart_Declaration=inline extern void Init_onlyOnce();  FctStart_Call=Init_onlyOnce();  FctInit=None  FctInit_Name=Init_Reset  FctInit_Declaration=inline extern void Init_Reset();  FctInit_Call=Init_Reset();  PinDigitalInput=[]  PinDigitalOutput=[]  AnalogueInput=[]
  Get the Pan [FCBEX1000.c]1 : dsPICdrivers/OTHERS/C Function Call  Tag=dsPIC_dsPIC_CFunctionCall  FctUpdate=Output Function  fctName='getTiltValue'  INPUT_SIZE=1  INPUT1=uint8  INPUT2=--  INPUT3=--  OUTPUT_SIZE=1  OUTPUT1=uint16  SampleTime=0.01  InputType=[ 2 ]  OutputType=[ 4 ]  FctDeclaration=extern uint16_T getTiltValue(uint8_T u1);  FctCall=%y1 = getTiltValue(%u1);  OrderingInOutPopup=None  FctStart=None  FctStart_Name=Init_onlyOnce  FctStart_Declaration=inline extern void Init_onlyOnce();  FctStart_Call=Init_onlyOnce();  FctInit=None  FctInit_Name=Init_Reset  FctInit_Declaration=inline extern void Init_Reset();  FctInit_Call=Init_Reset();  PinDigitalInput=[]  PinDigitalOutput=[]  AnalogueInput=[]
  Roll Compensation : Subsystem
  Set Camera to Home Position? [FCBEX1000.c]1 : dsPICdrivers/OTHERS/C Function Call  Tag=dsPIC_dsPIC_CFunctionCall  FctUpdate=Output Function  fctName='getGoHome'  INPUT_SIZE=1  INPUT1=--  INPUT2=--  INPUT3=--  OUTPUT_SIZE=1  OUTPUT1=uint8  SampleTime=0.01  InputType=[ ]  OutputType=[ 2 ]  FctDeclaration=extern uint8_T getGoHome();  FctCall=%y1 = getGoHome();  OrderingInOutPopup=None  FctStart=None  FctStart_Name=Init_onlyOnce  FctStart_Declaration=inline extern void Init_onlyOnce();  FctStart_Call=Init_onlyOnce();  FctInit=None  FctInit_Name=Init_Reset  FctInit_Declaration=inline extern void Init_Reset();  FctInit_Call=Init_Reset();  PinDigitalInput=[]  PinDigitalOutput=[]  AnalogueInput=[]
  Switch1 : Switch  Criteria=u2 > Threshold  Threshold=0.3  ZeroCross=off
  Terminator : Terminator
  Terminator1 : Terminator
  Terminator2 : Terminator
  "Tustin Lowpass, Auto Initial Condition1" : Subsystem  mask(Tustin1stOrderLowpassAutoInitialCondition){f=60, T=T}
      mask prompts: f "Lowpass Frequency"; T "Sample Time"
      mask help: Takes a 3db rolloff frequency (in Hz, NOT radians/s) and a sample time. Performs a symbolic Tustin conversion and implements in a discrete filter. The initial output of the filter is set by the first sample.
      mask Help: Enter the desired 3db rolloff frequency in Hz and the sample time. Initial conditions are sampled automatically.
      mask Display: fprintf('%.2f Hz lowpass',f)
  Zero Roll : Constant  Value=977  OutDataTypeStr=uint16
  Zero Tilt (max Tilt) : Constant  Value=1266  OutDataTypeStr=uint16
  Tilt_c (abs) : Outport
  Pan_c (abs) : Outport  Port=2
  Roll_c (abs) : Outport  Port=3
  wires:
  Set Camera to Home Position? [FCBEX1000.c]1/1 -> Get the Pan [FCBEX1000.c]/1, Get the Pan [FCBEX1000.c]1/1
  Euler/1 -> Demux1/1
  Demux1/3 -> Terminator/1
  "Tustin Lowpass, Auto Initial Condition1"/1(Out1) -> Gain2/1
  Demux1/1 -> Roll Compensation/1(Roll)
  Get the Pan [FCBEX1000.c]/1 -> Roll Compensation/2(Pan(abs)), Pan_c (abs)/1
  Demux1/2 -> "Tustin Lowpass, Auto Initial Condition1"/1(In1)
  Get the Pan [FCBEX1000.c]1/1 -> Add/1
  Add/1 -> Tilt_c (abs)/1
  Gain2/1 -> Convert to PWM3/1(" Angle(rad)")
  Currently No Roll  Comp/1 -> Roll Compensation/Enable, Switch1/2
  Switch1/1 -> Roll_c (abs)/1
  Roll Compensation/1(Roll Correction) -> Switch1/1
  Zero Roll/1 -> Switch1/3
  Zero Tilt (max Tilt)/1 -> Terminator1/1
  Convert to PWM3/1(PWM) -> Terminator2/1
  Constant/1 -> Add/3, Add/2

== system intgratedMCUSlugs/Update PWM Commands and Send Telemetry/PTZ Unit/Camera Track ==
  Euler : Inport
  Camera Location : Inport  Port=2
  Puav : Inport  Port=3
  ISR Location : Inport  Port=4
  Enable : EnablePort
  Convert to PWM2 : Subsystem  mask{slopem=mtilt, interceptb=btilt}
      mask prompts: slopem "Slope"; interceptb "Intercept"
  Convert to PWM4 : Subsystem  mask{slopem=mpan, interceptb=bpan}
      mask prompts: slopem "Slope"; interceptb "Intercept"
  Data Type Conversion9 : DataTypeConversion  OutDataTypeStr=single
  Get the Aide Pan [FCBEX1000c] : dsPICdrivers/OTHERS/C Function Call  Tag=dsPIC_dsPIC_CFunctionCall  FctUpdate=Output Function  fctName='getPanISRAide'  INPUT_SIZE=1  INPUT1=uint8  INPUT2=--  INPUT3=--  OUTPUT_SIZE=1  OUTPUT1=int16  SampleTime=.01  InputType=[ 2 ]  OutputType=[ 3 ]  FctDeclaration=extern int16_T getPanISRAide(uint8_T u1);  FctCall=%y1 = getPanISRAide(%u1);  OrderingInOutPopup=None  FctStart=None  FctStart_Name=Init_onlyOnce  FctStart_Declaration=inline extern void Init_onlyOnce();  FctStart_Call=Init_onlyOnce();  FctInit=None  FctInit_Name=Init_Reset  FctInit_Declaration=inline extern void Init_Reset();  FctInit_Call=Init_Reset();  PinDigitalInput=[]  PinDigitalOutput=[]  AnalogueInput=[]
  Get the Aide Tilt [FCBEX1000.c] : dsPICdrivers/OTHERS/C Function Call  Tag=dsPIC_dsPIC_CFunctionCall  FctUpdate=Output Function  fctName='getTiltISRAide'  INPUT_SIZE=1  INPUT1=uint8  INPUT2=--  INPUT3=--  OUTPUT_SIZE=1  OUTPUT1=int16  SampleTime=.01  InputType=[ 2 ]  OutputType=[ 3 ]  FctDeclaration=extern int16_T getTiltISRAide(uint8_T u1);  FctCall=%y1 = getTiltISRAide(%u1);  OrderingInOutPopup=None  FctStart=None  FctStart_Name=Init_onlyOnce  FctStart_Declaration=inline extern void Init_onlyOnce();  FctStart_Call=Init_onlyOnce();  FctInit=None  FctInit_Name=Init_Reset  FctInit_Declaration=inline extern void Init_Reset();  FctInit_Call=Init_Reset();  PinDigitalInput=[]  PinDigitalOutput=[]  AnalogueInput=[]
  LPF the Euler and Construct Matrix : Subsystem
  Normalize : Product  Inputs=*/
  Product1 : Product  Multiplication=Matrix(*)  RndMeth=Zero
  Product2 : Product  Multiplication=Matrix(*)  RndMeth=Zero
  Set Aides to Zero? [FCBEX1000.c] : dsPICdrivers/OTHERS/C Function Call  Tag=dsPIC_dsPIC_CFunctionCall  FctUpdate=Output Function  fctName='getGoHome'  INPUT_SIZE=1  INPUT1=--  INPUT2=--  INPUT3=--  OUTPUT_SIZE=1  OUTPUT1=uint8  SampleTime=0.01  InputType=[ ]  OutputType=[ 2 ]  FctDeclaration=extern uint8_T getGoHome();  FctCall=%y1 = getGoHome();  OrderingInOutPopup=None  FctStart=None  FctStart_Name=Init_onlyOnce  FctStart_Declaration=inline extern void Init_onlyOnce();  FctStart_Call=Init_onlyOnce();  FctInit=None  FctInit_Name=Init_Reset  FctInit_Declaration=inline extern void Init_Reset();  FctInit_Call=Init_Reset();  PinDigitalInput=[]  PinDigitalOutput=[]  AnalogueInput=[]
  Subtract1 : Sum
  Subtract2 : Sum  Inputs=-+
  Sum : Sum  Inputs=|++  OutDataTypeStr=uint16
  Sum1 : Sum  Inputs=++|  OutDataTypeStr=uint16
  Transpose1 : dspmtrx3/Transpose  Hermitian=off  overflowFlag=off
  Vector Norm : SLUGS_Library/Vector Norm
  Zero Roll : Constant  Value=977  OutDataTypeStr=uint16
  "[a b c]" : Demux  Outputs=3
  dsPIC_asin : SLUGS_Library/dsPIC_asin
  dsPIC_atan2 : SLUGS_Library/dsPIC_atan2
  Tilt_c (abs) : Outport
  Pan_c (abs) : Outport  Port=2
  Roll_c(abs) : Outport  Port=3  InitialOutput=977
  wires:
  Subtract2/1 -> Normalize/1, Vector Norm/1
  Subtract1/1 -> Subtract2/1
  dsPIC_atan2/1 -> Convert to PWM4/1(" Angle(rad)")
  "[a b c]"/1 -> dsPIC_atan2/2
  "[a b c]"/2 -> dsPIC_atan2/1
  "[a b c]"/3 -> dsPIC_asin/1
  Product2/1 -> "[a b c]"/1
  Normalize/1 -> Product2/2
  Vector Norm/1 -> Normalize/2
  Product1/1 -> Subtract1/1  "Tgb * cor_b"
  Puav/1 -> Subtract1/2  "Xac"
  ISR Location/1 -> Subtract2/2  "Xt"
  Camera Location/1 -> Product1/2
  Zero Roll/1 -> Roll_c(abs)/1
  Transpose1/1 -> Product1/1
  Euler/1 -> LPF the Euler and Construct Matrix/1(Euler)
  LPF the Euler and Construct Matrix/1(Rfg2b) -> Data Type Conversion9/1
  Data Type Conversion9/1 -> Transpose1/1, Product2/1  "Rfg2b"
  dsPIC_asin/1 -> Convert to PWM2/1(" Angle(rad)")
  Sum/1 -> Pan_c (abs)/1
  Convert to PWM4/1(PWM) -> Sum/1
  Get the Aide Pan [FCBEX1000c]/1 -> Sum/2
  Sum1/1 -> Tilt_c (abs)/1
  Convert to PWM2/1(PWM) -> Sum1/2
  Get the Aide Tilt [FCBEX1000.c]/1 -> Sum1/1
  Set Aides to Zero? [FCBEX1000.c]/1 -> Get the Aide Pan [FCBEX1000c]/1, Get the Aide Tilt [FCBEX1000.c]/1

== system intgratedMCUSlugs/Update PWM Commands and Send Telemetry/PTZ Unit/Pan ==
  OC : Inport
  Angle Conversion : aerolibconvert2/Angle Conversion  IU=rad  OU=deg
  Convert to OC1 : Subsystem  mask{slopem=mPWMpan, interceptb=bPWMpan}
      mask prompts: slopem "Slope"; interceptb "Intercept"
  Data Type Conversion1 : DataTypeConversion  OutDataTypeStr=int16
  Gain : Gain  Gain=10
  0.1Deg : Outport
  wires:
  Data Type Conversion1/1 -> 0.1Deg/1
  OC/1 -> Convert to OC1/1(" OC(abs)")
  Gain/1 -> Data Type Conversion1/1
  Angle Conversion/1 -> Gain/1
  Convert to OC1/1(Angle (rad)) -> Angle Conversion/1

== system intgratedMCUSlugs/Update PWM Commands and Send Telemetry/PTZ Unit/Tilt ==
  OC : Inport
  Angle Conversion : aerolibconvert2/Angle Conversion  IU=rad  OU=deg
  Convert to OC1 : Subsystem  mask{slopem=mPWMtilt, interceptb=bPWMtilt}
      mask prompts: slopem "Slope"; interceptb "Intercept"
  Data Type Conversion1 : DataTypeConversion  OutDataTypeStr=int16
  Gain : Gain  Gain=10
  0.1Deg : Outport
  wires:
  Convert to OC1/1(Angle (rad)) -> Angle Conversion/1
  Angle Conversion/1 -> Gain/1
  Gain/1 -> Data Type Conversion1/1
  OC/1 -> Convert to OC1/1(" OC(abs)")
  Data Type Conversion1/1 -> 0.1Deg/1

== system intgratedMCUSlugs/Inner Loop/ Navigation/L1 Output Feedback Controller With  Projection Operator/Control  Law/Compute Coef ==
  a : Inport
  Enable : EnablePort
  -T : Gain  Gain=-apSampleTime  SampleTime=apSampleTime
  1-c : Sum  Inputs=-+  OutDataTypeStr=single  SampleTime=apSampleTime
  Constant : Constant
  dsPIC_exp : SLUGS_Library/dsPIC_exp
  b : Outport
  c : Outport  Port=2
  wires:
  -T/1 -> dsPIC_exp/1
  dsPIC_exp/1 -> 1-c/1, c/1  "c"
  Constant/1 -> 1-c/2
  1-c/1 -> b/1
  a/1 -> -T/1

== system intgratedMCUSlugs/Inner Loop/ Navigation/L1 Output Feedback Controller With  Projection Operator/Control  Law/Detect Change ==
  Data : Inport
  Abs1 : Abs  SampleTime=apSampleTime
  Difference1 : simulink/Discrete/Difference  ICPrevInput=0.0  InputProcessing=Inherited  OutMin=[]  OutMax=[]  OutDataType=sfix(16)  OutScaling=2^-10  DoSatur=off
  Saturation1 : Saturate  UpperLimit=1  LowerLimit=0  SampleTime=apSampleTime
  change? : Outport
  wires:
  Difference1/1 -> Abs1/1
  Abs1/1 -> Saturation1/1
  Data/1 -> Difference1/1
  Saturation1/1 -> change?/1

== system intgratedMCUSlugs/Inner Loop/ Navigation/L1 Output Feedback Controller With  Projection Operator/Projection Operator/Enabled Subsystem ==
  In1 : Inport
  Enable : EnablePort
  Out1 : Outport
  wires:
  In1/1 -> Out1/1

== system intgratedMCUSlugs/Inner Loop/ Navigation/L1 Output Feedback Controller With  Projection Operator/Projection Operator/Enabled Subsystem1 ==
  y : Inport
  f_the : Inport  Port=2
  grad : Inport  Port=3
  Enable : EnablePort
  Constant : Constant  OutDataTypeStr=single
  Divide1 : Product  OutDataTypeStr=single
  Divide2 : Product  OutDataTypeStr=single
  Sign : Signum
  Subtract : Sum  Inputs=+-  OutDataTypeStr=single
  Out1 : Outport
  wires:
  Divide1/1 -> Subtract/2
  grad/1 -> Sign/1
  Sign/1 -> Divide1/2
  Constant/1 -> Subtract/1
  f_the/1 -> Divide1/1
  Subtract/1 -> Divide2/2
  y/1 -> Divide2/1
  Divide2/1 -> Out1/1

== system intgratedMCUSlugs/Inner Loop/ Navigation/L1 Output Feedback Controller With  Projection Operator/Projection Operator/F(theta) ==
  Theta Max : Inport
  Eps 0 : Inport  Port=2
  Theta : Inport  Port=3
  Constant : Constant  Value=2  OutDataTypeStr=single
  Divide : Product  OutDataTypeStr=single
  Divide1 : Product  OutDataTypeStr=single
  Divide2 : Product  OutDataTypeStr=single
  Divide3 : Product  Inputs=*/  OutDataTypeStr=single
  Divide4 : Product  Inputs=/**  OutDataTypeStr=single
  Subtract : Sum  Inputs=+-  OutDataTypeStr=single
  "Theta " : InportShadow  Port=3
  f_theta : Outport
  dif_f_theta : Outport  Port=2
  wires:
  Theta/1 -> Divide/1, Divide/2
  Theta Max/1 -> Divide1/2, Divide1/1
  Divide/1 -> Subtract/1
  Divide1/1 -> Subtract/2, Divide2/1
  Eps 0/1 -> Divide2/2
  Subtract/1 -> Divide3/1
  Divide2/1 -> Divide3/2, Divide4/1
  Divide3/1 -> f_theta/1
  Constant/1 -> Divide4/3
  "Theta "/1 -> Divide4/2
  Divide4/1 -> dif_f_theta/1

== system intgratedMCUSlugs/Inner Loop/ Navigation/L1 Output Feedback Controller With  Projection Operator/State Predictor/Compute Coef ==
  a : Inport
  Enable : EnablePort
  -T : Gain  Gain=-apSampleTime  SampleTime=apSampleTime
  1-c : Sum  Inputs=-+  OutDataTypeStr=single
  Constant : Constant
  dsPIC_exp : SLUGS_Library/dsPIC_exp
  b : Outport
  c : Outport  Port=2
  wires:
  a/1 -> -T/1
  1-c/1 -> b/1
  Constant/1 -> 1-c/2
  dsPIC_exp/1 -> c/1, 1-c/1  "c"
  -T/1 -> dsPIC_exp/1

== system intgratedMCUSlugs/Inner Loop/ Navigation/L1 Output Feedback Controller With  Projection Operator/State Predictor/Detect Change ==
  Data : Inport
  Abs1 : Abs  SampleTime=apSampleTime
  Difference1 : simulink/Discrete/Difference  ICPrevInput=0.0  InputProcessing=Inherited  OutMin=[]  OutMax=[]  OutDataType=sfix(16)  OutScaling=2^-10  DoSatur=off
  Saturation1 : Saturate  UpperLimit=1  LowerLimit=0  SampleTime=apSampleTime
  change? : Outport
  wires:
  Saturation1/1 -> change?/1
  Data/1 -> Difference1/1
  Abs1/1 -> Saturation1/1
  Difference1/1 -> Abs1/1

== system intgratedMCUSlugs/Inner Loop/ Navigation/L1 Output Feedback Controller With  Projection Operator/Trapezoidal Integrator/Protect NaNs ==
  In1 : Inport
  Integer Delay3 : Delay  DelayLength=1  InputProcessing=Inherited  SampleTime=T
  Relational Operator2 : RelationalOperator  Operator===  OutDataTypeStr=uint(8)
  Switch3 : Switch  Criteria=u2 > Threshold  Threshold=0.3  SampleTime=.01
  Out1 : Outport
  wires:
  Relational Operator2/1 -> Switch3/2
  In1/1 -> Switch3/1, Relational Operator2/1, Relational Operator2/2
  Switch3/1 -> Integer Delay3/1, Out1/1
  Integer Delay3/1 -> Switch3/3

== system intgratedMCUSlugs/Inner Loop/ Navigation/L1 Output Feedback Controller With  Projection Operator/Trapezoidal Integrator/Protect NaNs1 ==
  In1 : Inport
  Integer Delay3 : Delay  DelayLength=1  InputProcessing=Inherited  SampleTime=T
  Relational Operator2 : RelationalOperator  Operator===  OutDataTypeStr=uint(8)
  Switch3 : Switch  Criteria=u2 > Threshold  Threshold=0.3  SampleTime=.01
  Out1 : Outport
  wires:
  Integer Delay3/1 -> Switch3/3
  Switch3/1 -> Out1/1, Integer Delay3/1
  In1/1 -> Relational Operator2/2, Relational Operator2/1, Switch3/1
  Relational Operator2/1 -> Switch3/2

== system intgratedMCUSlugs/Position and Attitude Filter/Attitude Complimentary Filter COG/3D Filter/Filter1 ==
  In1 : Inport
  Discrete Zero-Pole : DiscreteZeroPole  Zeros=zerosd  Poles=polesd  Gain=gaind  SampleTime=SampleTime
  Out1 : Outport
  wires:
  Discrete Zero-Pole/1 -> Out1/1
  In1/1 -> Discrete Zero-Pole/1

== system intgratedMCUSlugs/Position and Attitude Filter/Attitude Complimentary Filter COG/3D Filter/Filter2 ==
  In1 : Inport
  Discrete Zero-Pole : DiscreteZeroPole  Zeros=zerosd  Poles=polesd  Gain=gaind  SampleTime=SampleTime
  Out1 : Outport
  wires:
  In1/1 -> Discrete Zero-Pole/1
  Discrete Zero-Pole/1 -> Out1/1

== system intgratedMCUSlugs/Position and Attitude Filter/Attitude Complimentary Filter COG/3D Filter/Filter3 ==
  In1 : Inport
  Discrete Zero-Pole : DiscreteZeroPole  Zeros=zerosd  Poles=polesd  Gain=gaind  SampleTime=SampleTime
  Out1 : Outport
  wires:
  Discrete Zero-Pole/1 -> Out1/1
  In1/1 -> Discrete Zero-Pole/1

== system intgratedMCUSlugs/Position and Attitude Filter/Attitude Complimentary Filter COG/Normalize Vector1/Norm ==
  Vector : Inport
  Subsystem2 : Subsystem  AncestorBlock=SLUGS_Library/Subsystem1
  Subsystem3 : Subsystem  AncestorBlock=SLUGS_Library/Subsystem3
  Norm : Outport
  wires:
  Subsystem3/1(x dot y) -> Subsystem2/1(x)
  Vector/1 -> Subsystem3/2(y), Subsystem3/1(x)
  Subsystem2/1(sqrt(x)) -> Norm/1

== system intgratedMCUSlugs/Position and Attitude Filter/Attitude Complimentary Filter COG/Normalize Vector2/Norm ==
  Vector : Inport
  Subsystem2 : Subsystem  AncestorBlock=SLUGS_Library/Subsystem1
  Subsystem3 : Subsystem  AncestorBlock=SLUGS_Library/Subsystem3
  Norm : Outport
  wires:
  Subsystem2/1(sqrt(x)) -> Norm/1
  Vector/1 -> Subsystem3/1(x), Subsystem3/2(y)
  Subsystem3/1(x dot y) -> Subsystem2/1(x)

== system intgratedMCUSlugs/Position and Attitude Filter/Compute GS Location/Geod2ECEF1/eccentricity^2 ==
  " " : Product  OutDataTypeStr=single  SaturateOnIntegerOverflow=on  InputSameDT=on
  Re=equatorial radius1 : Constant  Value=Re  OutDataTypeStr=single
  Rp=polar radius : Constant  Value=Rp  OutDataTypeStr=single
  Sum5 : Sum  Inputs=|+-  SaturateOnIntegerOverflow=on  InputSameDT=on  OutDataTypeStr=Inherit: Same as first input
  const2 : Constant  OutDataTypeStr=single
  e^1 : Product  Inputs=*/  OutDataTypeStr=single  SaturateOnIntegerOverflow=on  InputSameDT=on
  e^2 : Outport
  wires:
  Sum5/1 -> e^2/1
  " "/1 -> Sum5/2
  e^1/1 -> " "/1, " "/2
  const2/1 -> Sum5/1
  Rp=polar radius/1 -> e^1/1
  Re=equatorial radius1/1 -> e^1/2

== system intgratedMCUSlugs/Position and Attitude Filter/Geod2LTP1/ECEF2LTP (UEN)/From Body to Universal1 ==
  long : Inport
  lat : Inport  Port=2
  Mux : Mux  Inputs=2
  Reshape 9x1->3x1 : Reshape  OutputDimensionality=Customize  OutputDimensions=[3,3]
  Rotation Matrix from Long//Lat : Subsystem
      mask Type: Vector Transformation
      mask Description: Vector Transformation
      mask Display: disp('axis')
  DCM : Outport
  wires:
  Reshape 9x1->3x1/1 -> DCM/1
  Rotation Matrix from Long//Lat/1(DCM) -> Reshape 9x1->3x1/1
  Mux/1 -> Rotation Matrix from Long//Lat/1(long lat)
  long/1 -> Mux/1
  lat/1 -> Mux/2

== system intgratedMCUSlugs/Position and Attitude Filter/Geod2LTP1/Geod2ECEF1/eccentricity^2 ==
  " " : Product  OutDataTypeStr=single  SaturateOnIntegerOverflow=on  InputSameDT=on
  Re=equatorial radius1 : Constant  Value=Re  OutDataTypeStr=single
  Rp=polar radius : Constant  Value=Rp  OutDataTypeStr=single
  Sum5 : Sum  Inputs=|+-  SaturateOnIntegerOverflow=on  InputSameDT=on  OutDataTypeStr=Inherit: Same as first input
  const2 : Constant  OutDataTypeStr=single
  e^1 : Product  Inputs=*/  OutDataTypeStr=single  SaturateOnIntegerOverflow=on  InputSameDT=on
  e^2 : Outport
  wires:
  Sum5/1 -> e^2/1
  " "/1 -> Sum5/2
  e^1/1 -> " "/1, " "/2
  const2/1 -> Sum5/1
  Rp=polar radius/1 -> e^1/1
  Re=equatorial radius1/1 -> e^1/2
